simulink model "validation"  (R2017b)
settings: Solver=VariableStepAuto  StartTime=0.0  StopTime=9  RelTol=1e-3
values from neighbouring files (symbols this model uses):
  Kd = Kc*Td    (= 8.9468779124)    [identification.m]
  Ki = Kc/Ti    (= 8387.69804287)    [identification.m]
  Kp = Kc    (= 559.179869525)    [identification.m]
libraries: cstblocks x5
settings Model: Creator=Enrique  LastModifiedBy=Enrique

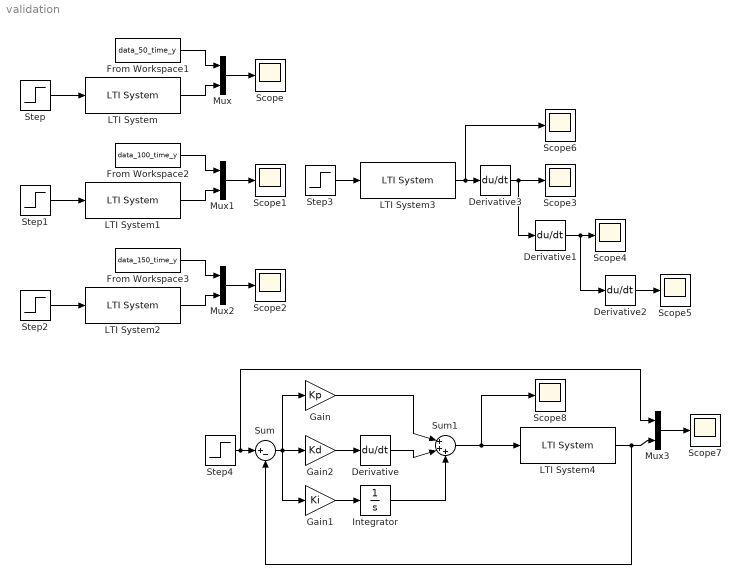
== system validation ==
  Derivative{,1..3} (4 alike) : Derivative
  From Workspace1 : FromWorkspace  VariableName=data_50_time_y  SampleTime=0
  From Workspace2 : FromWorkspace  VariableName=data_100_time_y  SampleTime=0
  From Workspace3 : FromWorkspace  VariableName=data_150_time_y  SampleTime=0
  Gain : Gain  Gain=Kp
  Gain1 : Gain  Gain=Ki
  Gain2 : Gain  Gain=Kd
  Integrator : Integrator
  LTI System{,1..4} (5 alike) : cstblocks/LTI System  sys=sys  IC=[]
  Mux{,1..3} (4 alike) : Mux  Inputs=2
  Scope{,1..8} (9 alike) : Scope
  Step : Step  Time=0  After=50  SampleTime=0
  Step1 : Step  Time=0  After=100  SampleTime=0
  Step2 : Step  Time=0  After=150  SampleTime=0
  Step3 : Step  Time=0  SampleTime=0
  Step4 : Step  Time=0  After=40  SampleTime=0
  Sum : Sum  Inputs=|+-
  Sum1 : Sum  Inputs=|+++
  wires:
  Step/1 -> LTI System/1
  Mux/1 -> Scope/1
  LTI System/1 -> Mux/2
  From Workspace1/1 -> Mux/1
  From Workspace2/1 -> Mux1/1
  LTI System1/1 -> Mux1/2
  Mux1/1 -> Scope1/1
  Step1/1 -> LTI System1/1
  From Workspace3/1 -> Mux2/1
  LTI System2/1 -> Mux2/2
  Mux2/1 -> Scope2/1
  Step2/1 -> LTI System2/1
  LTI System3/1 -> Scope6/1, Derivative3/1
  Derivative3/1 -> Scope3/1, Derivative1/1
  Derivative1/1 -> Scope4/1, Derivative2/1
  Step3/1 -> LTI System3/1
  Derivative2/1 -> Scope5/1
  Mux3/1 -> Scope7/1
  LTI System4/1 -> Sum/2, Mux3/2
  Sum/1 -> Gain/1, Gain1/1, Gain2/1
  Gain2/1 -> Derivative/1
  Gain1/1 -> Integrator/1
  Derivative/1 -> Sum1/2
  Gain/1 -> Sum1/1
  Integrator/1 -> Sum1/3
  Sum1/1 -> Scope8/1, LTI System4/1
  Step4/1 -> Mux3/1, Sum/1
